simulink subsystem "HallSensor1"  (R2023a)
settings: Solver=VariableStepAuto  StartTime=0.0  StopTime=10.0  RelTol=1e-3
settings Model: Creator=stude  LastModifiedBy=mehra

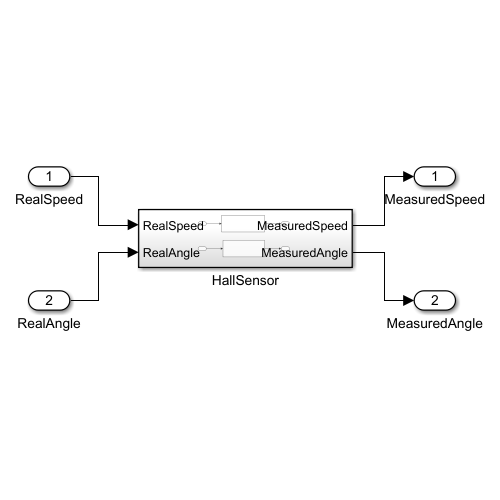
[thumbnail: Simulink's stored preview of the top-level diagram]
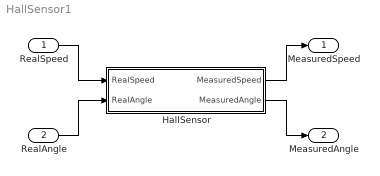
== system HallSensor1 ==
  RealSpeed : Inport
  RealAngle : Inport  Port=2
  HallSensor : Subsystem
  MeasuredSpeed : Outport
  MeasuredAngle : Outport  Port=2
  wires:
  RealSpeed/1 -> HallSensor/1(RealSpeed)
  RealAngle/1 -> HallSensor/2(RealAngle)
  HallSensor/1(MeasuredSpeed) -> MeasuredSpeed/1
  HallSensor/2(MeasuredAngle) -> MeasuredAngle/1

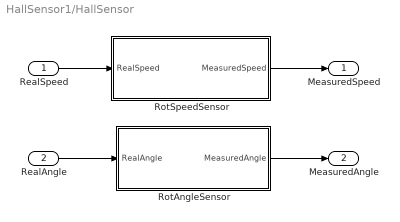
== system HallSensor1/HallSensor ==
  RealSpeed : Inport
  RealAngle : Inport  Port=2
  RotAngleSensor : Subsystem
  RotSpeedSensor : Subsystem
  MeasuredSpeed : Outport
  MeasuredAngle : Outport  Port=2
  wires:
  RealSpeed/1 -> RotSpeedSensor/1(RealSpeed)
  RealAngle/1 -> RotAngleSensor/1(RealAngle)
  RotAngleSensor/1(MeasuredAngle) -> MeasuredAngle/1
  RotSpeedSensor/1(MeasuredSpeed) -> MeasuredSpeed/1

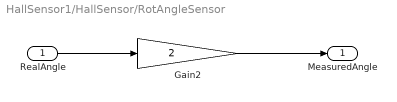
== system HallSensor1/HallSensor/RotAngleSensor ==
  RealAngle : Inport
  Gain2 : Gain  Gain=2
  MeasuredAngle : Outport
  wires:
  RealAngle/1 -> Gain2/1
  Gain2/1 -> MeasuredAngle/1

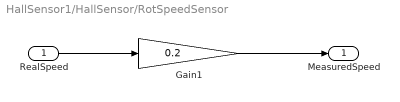
== system HallSensor1/HallSensor/RotSpeedSensor ==
  RealSpeed : Inport
  Gain1 : Gain  Gain=0.2
  MeasuredSpeed : Outport
  wires:
  RealSpeed/1 -> Gain1/1
  Gain1/1 -> MeasuredSpeed/1
